simulink model "io"  (R2017b)
settings: Solver=VariableStepAuto  StartTime=0.0  StopTime=10.0  RelTol=1e-3
settings Model: Creator=yaakovazat  LastModifiedBy=yaakovazat

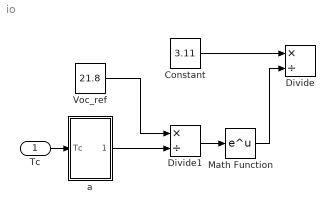
== system io ==
  Tc : Inport
  Constant : Constant  Value=3.11
  Divide : Product  Inputs=*/
  Divide1 : Product  Inputs=*/
  Math Function : Math  SaturateOnIntegerOverflow=on
  Voc_ref : Constant  Value=21.8
  a : Subsystem
  wires:
  Tc/1 -> a/1(Tc)
  a/1(Out1) -> Divide1/2
  Voc_ref/1 -> Divide1/1
  Divide1/1 -> Math Function/1
  Constant/1 -> Divide/1
  Math Function/1 -> Divide/2

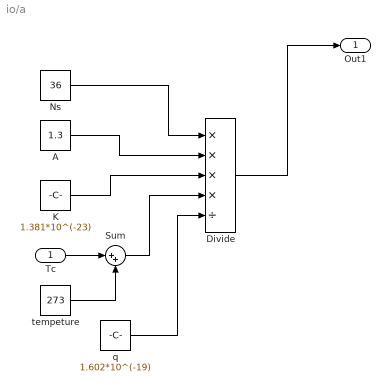
== system io/a ==
  Tc : Inport
  A : Constant  Value=1.3
  Divide : Product  Inputs=****/
  K : Constant  Value=1.381*10^(-23)
  Ns : Constant  Value=36
  Sum : Sum  Inputs=|++
  q : Constant  Value=1.602*10^(-19)
  tempeture : Constant  Value=273
  Out1 : Outport
  wires:
  q/1 -> Divide/5
  Sum/1 -> Divide/4
  Ns/1 -> Divide/1
  K/1 -> Divide/3
  A/1 -> Divide/2
  tempeture/1 -> Sum/2
  Tc/1 -> Sum/1
  Divide/1 -> Out1/1
